simulink model "plant_bike_lin"  (R2022a)
settings: Solver=VariableStepAuto  StartTime=0.0  StopTime=10.0  RelTol=1e-3
values from neighbouring files (symbols this model uses):
  x_0 = block.DialogPrm(7).Data    [msfun_plant_bikeModel.m]
undefined symbols (not defined in the file or in its folder): K_error_weighted, params, W_driver, W_drivetrain, w_in_gain
libraries: cstblocks x10, RCTblocks x4
settings Model: Creator=Jonas  LastModifiedBy=Jonas
settings DataIOCC: SaveOutput=off  SaveTime=off
settings GRTTargetCC: CombineOutputUpdateFcns=off  MatFileLogging=off

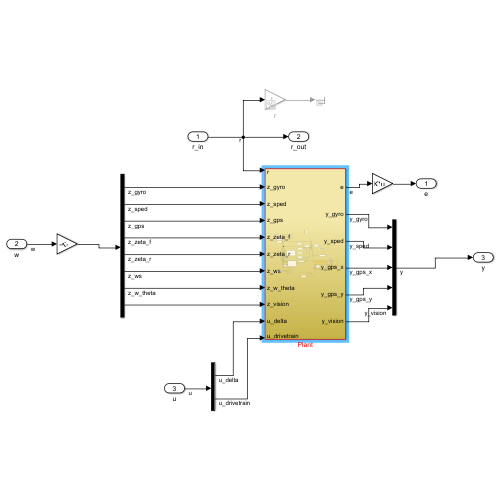
[thumbnail: Simulink's stored preview of the top-level diagram]
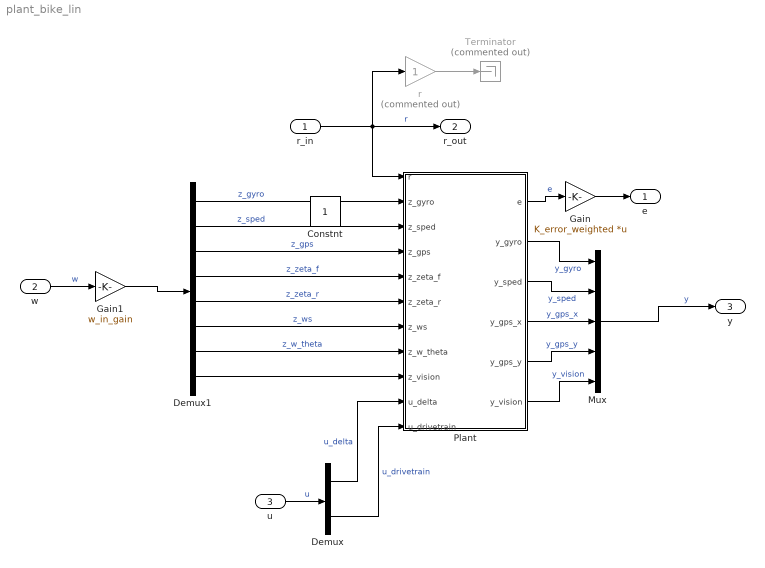
== system plant_bike_lin ==
  r_in : Inport  OutDataTypeStr=double  PortDimensions=6
  w : Inport  Port=2  OutDataTypeStr=double  SampleTime=0
  u : Inport  Port=3  OutDataTypeStr=double  PortDimensions=2  SampleTime=0
  Demux : Demux  Outputs=2
  Demux1 : Demux  Outputs=8
  Gain : Gain  Gain=K_error_weighted  Multiplication=Matrix(K*u)
  Gain1 : Gain  Gain=w_in_gain
  Mux : Mux  Inputs=5
  Plant : Subsystem
  Terminator : Terminator  Commented=on
  r : Gain  Commented=on
  e : Outport  OutDataTypeStr=double  SampleTime=0
  r_out : Outport  Port=2
  y : Outport  Port=3  OutDataTypeStr=double  SampleTime=0
  Constnt : Constant  IOType=siggen
  wires:
  Mux/1 -> y/1  "y"
  w/1 -> Gain1/1  "w"
  Demux/1 -> Plant/10(u_delta)  "u_delta"
  Plant/1(e) -> Gain/1  "e"
  Plant/5(y_gps_y) -> Mux/4  "y_gps_y"
  Plant/4(y_gps_x) -> Mux/3  "y_gps_x"
  Plant/3(y_sped) -> Mux/2  "y_sped"
  Demux/2 -> Plant/11(u_drivetrain)  "u_drivetrain"
  Plant/2(y_gyro) -> Mux/1  "y_gyro"
  u/1 -> Demux/1  "u"
  r_in/1 -> r/1, Plant/1(r), r_out/1  "r"
  r/1 -> Terminator/1
  Gain/1 -> e/1
  Demux1/1 -> Plant/2(z_gyro)  "z_gyro"
  Demux1/2 -> Plant/3(z_sped)  "z_sped"
  Demux1/7 -> Plant/8(z_w_theta)  "z_w_theta"
  Demux1/5 -> Plant/6(z_zeta_r)  "z_zeta_r"
  Demux1/4 -> Plant/5(z_zeta_f)  "z_zeta_f"
  Demux1/3 -> Plant/4(z_gps)  "z_gps"
  Demux1/6 -> Plant/7(z_ws)  "z_ws"
  Gain1/1 -> Demux1/1
  Plant/6(y_vision) -> Mux/5  "y_vision"
  Demux1/8 -> Plant/9(z_vision)

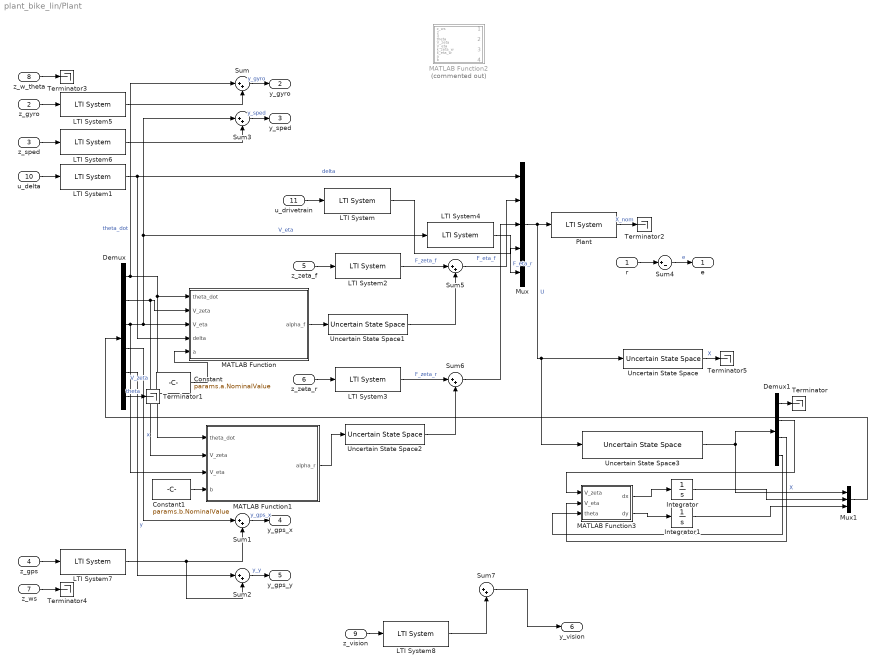
== system plant_bike_lin/Plant ==
  r : Inport
  z_gyro : Inport  Port=2
  z_sped : Inport  Port=3
  z_gps : Inport  Port=4
  z_zeta_f : Inport  Port=5
  z_zeta_r : Inport  Port=6
  z_ws : Inport  Port=7
  z_w_theta : Inport  Port=8
  z_vision : Inport  Port=9
  u_delta : Inport  Port=10
  u_drivetrain : Inport  Port=11
  Constant : Constant  Value=params.a.NominalValue
  Constant1 : Constant  Value=params.b.NominalValue
  Demux : Demux  Outputs=6
  Demux1 : Demux
  Integrator : Integrator
  Integrator1 : Integrator
  LTI System : cstblocks/LTI System  sys=W_driver * W_drivetrain  IC=[]
  LTI System1 : cstblocks/LTI System  sys=W_driver  IC=[]
  LTI System2 : cstblocks/LTI System  sys=W_zeta_f  IC=[]
  LTI System3 : cstblocks/LTI System  sys=W_zeta_r  IC=[]
  LTI System4 : cstblocks/LTI System  sys=W_ws  IC=[]
  LTI System5 : cstblocks/LTI System  sys=W_gyro  IC=[]
  LTI System6 : cstblocks/LTI System  sys=W_sped  IC=[]
  LTI System7 : cstblocks/LTI System  sys=W_gps  IC=[]
  LTI System8 : cstblocks/LTI System  sys=W_vision  IC=[]
  MATLAB Function : MATLAB Function  TreatAsAtomicUnit=on
  MATLAB Function1 : MATLAB Function  TreatAsAtomicUnit=on
  MATLAB Function2 : MATLAB Function  Commented=on  TreatAsAtomicUnit=on
  MATLAB Function3 : MATLAB Function  TreatAsAtomicUnit=on
  Mux : Mux  Inputs=5
  Mux1 : Mux  Inputs=3
  Plant : cstblocks/LTI System  sys=sys_nom  IC=[]
  Sum{,1..3,5..7} (7 alike) : Sum  Inputs=|++
  Sum4 : Sum  Inputs=|+-
  Terminator{,1..5} (6 alike) : Terminator
  Uncertain State Space : RCTblocks/Uncertain State Space  Tag=USS  USystem=sys_plant_u  UValue=[]  X0=x_0  uX0=[]
      settings: SourceProductBaseCode=RC
  Uncertain State Space1 : RCTblocks/Uncertain State Space  Tag=USS  USystem=params.c_f  UValue=[]  X0=[]  uX0=[]
      settings: SourceProductBaseCode=RC
  Uncertain State Space2 : RCTblocks/Uncertain State Space  Tag=USS  USystem=params.c_f  UValue=[]  X0=[]  uX0=[]
      settings: SourceProductBaseCode=RC
  Uncertain State Space3 : RCTblocks/Uncertain State Space  Tag=USS  USystem=sys_plant_u_local  UValue=[]  X0=x_0([1:3,6])  uX0=[]
      settings: SourceProductBaseCode=RC
  e : Outport
  y_gyro : Outport  Port=2
  y_sped : Outport  Port=3
  y_gps_x : Outport  Port=4
  y_gps_y : Outport  Port=5
  y_vision : Outport  Port=6
  wires:
  Uncertain State Space2/1 -> Sum6/2
  MATLAB Function/1(alpha_f) -> Uncertain State Space1/1
  Uncertain State Space1/1 -> Sum5/2
  MATLAB Function1/1(alpha_r) -> Uncertain State Space2/1
  z_sped/1 -> LTI System6/1
  Sum4/1 -> e/1  "e"
  Demux/6 -> Terminator1/1  "theta"
  z_zeta_r/1 -> LTI System3/1
  LTI System3/1 -> Sum6/1  "F_zeta_r"
  Sum3/1 -> y_sped/1  "y_sped"
  z_zeta_f/1 -> LTI System2/1
  Sum1/1 -> y_gps_x/1  "y_gps_x"
  z_gyro/1 -> LTI System5/1
  Sum2/1 -> y_gps_y/1  "y_y"
  u_drivetrain/1 -> LTI System/1
  LTI System5/1 -> Sum/2
  Demux/5 -> Sum2/1  "y"
  LTI System2/1 -> Sum5/1  "F_zeta_f"
  LTI System6/1 -> Sum3/2
  Plant/1 -> Terminator2/1  "X_nom"
  z_w_theta/1 -> Terminator3/1
  z_gps/1 -> LTI System7/1
  z_ws/1 -> Terminator4/1
  Demux/4 -> Sum1/1  "x"
  r/1 -> Sum4/1
  Sum/1 -> y_gyro/1  "y_gyro"
  Demux/3 -> Sum3/1, LTI System4/1, MATLAB Function/3(V_eta), MATLAB Function1/3(V_eta)  "V_eta"
  u_delta/1 -> LTI System1/1
  Mux/1 -> Plant/1, Uncertain State Space3/1, Uncertain State Space/1  "U"
  LTI System7/1 -> Sum2/2, Sum1/2
  Demux/2 -> MATLAB Function1/2(V_zeta), MATLAB Function/2(V_zeta)  "V_zeta"
  Demux/1 -> MATLAB Function/1(theta_dot), MATLAB Function1/1(theta_dot), Sum/1  "theta_dot"
  LTI System1/1 -> Mux/1, MATLAB Function/4(delta)  "delta"
  Constant/1 -> MATLAB Function/5(a)
  Constant1/1 -> MATLAB Function1/4(b)
  Sum7/1 -> y_vision/1
  LTI System8/1 -> Sum7/2
  z_vision/1 -> LTI System8/1
  Sum5/1 -> Mux/2
  Sum6/1 -> Mux/3
  LTI System4/1 -> Mux/5  "F_eta_r"
  LTI System/1 -> Mux/4  "F_eta_f"
  Mux1/1 -> Demux/1
  MATLAB Function3/1(dx) -> Integrator/1
  MATLAB Function3/2(dy) -> Integrator1/1
  Integrator1/1 -> Mux1/3
  Integrator/1 -> Mux1/2
  Uncertain State Space3/1 -> Mux1/1, Demux1/1  "X"
  Demux1/2 -> MATLAB Function3/1(V_zeta)
  Demux1/3 -> MATLAB Function3/2(V_eta)
  Demux1/4 -> MATLAB Function3/3(theta)
  Demux1/1 -> Terminator/1
  Uncertain State Space/1 -> Terminator5/1  "X"

== matlab function plant_bike_lin/Plant/MATLAB Function1 ==
  data: theta_dot input; V_zeta input; alpha_r output; V_eta input; b input
function alpha_r = rear_slip_angle(theta_dot,V_zeta,V_eta,b)

alpha_r = (b * theta_dot + V_zeta) / V_eta;

== matlab function plant_bike_lin/Plant/MATLAB Function ==
  data: theta_dot input; V_zeta input; alpha_f output; V_eta input; delta input; a input
function alpha_f = front_slip_angle(theta_dot,V_zeta,V_eta, delta, a)

alpha_f = delta - (a * theta_dot + V_zeta) / V_eta;

== matlab function plant_bike_lin/Plant/MATLAB Function2 ==
  data: z_ws input; F_zeta_f output; z_w_theta input; k_ws_mag input; theta input; V_zeta input; V_eta input; k_zeta_w input; k_eta_w input; a input; b input; F_zeta_r output; F_eta_f output; F_eta_r output
function [F_zeta_f, F_zeta_r, F_eta_f, F_eta_r] = wind_resistance(z_ws, z_w_theta, k_ws_mag, theta, V_zeta, V_eta, k_zeta_w, k_eta_w, a, b)

    V_x = V_eta * cos(theta) - V_zeta * sin(theta);
    V_y = V_zeta * cos(theta) + V_eta * sin(theta);
    
    F_x = z_ws *

== matlab function plant_bike_lin/Plant/MATLAB Function3 ==
  data: V_zeta input; dx output; V_eta input; theta input; dy output
function [dx,dy] = fcn(V_zeta,V_eta,theta)

dx = -V_zeta * sin(theta) + V_eta * cos(theta);
dy = V_zeta * cos(theta) + V_eta * sin(theta);
